simulink model "CCR_DIAM4100_model"  (R2023a)
settings: Solver=FixedStepAuto  StartTime=0.0  StopTime=1  RelTol=1e-3
values from neighbouring files (symbols this model uses):
  DIAM4100 = evalin('base', 'DIAM4100')    [DIAM4100_applyModelParameters.m]    (also in DIAM4100_simParams.m = cfg; DIAM4100_tuneKiSweep.m; DIAM4100_validateControl.m)
undefined symbols (not defined in the file or in its folder): D1, lagging, pulse
libraries: spsThyristorLib x2, spsACVoltageSourceLib x1, spsCurrentMeasurementLib x1, slpidlib x1, spsLinearTransformerLib x1, spsPLLLib x1, spsPulseGeneratorThyristor6PulseLib x1, spsRMSLib x1, spsSeriesRLCBranchLib x1, spsVoltageMeasurementLib x1, sps_lib x1
settings Model: Creator=KSSS  LastModifiedBy=KSSS

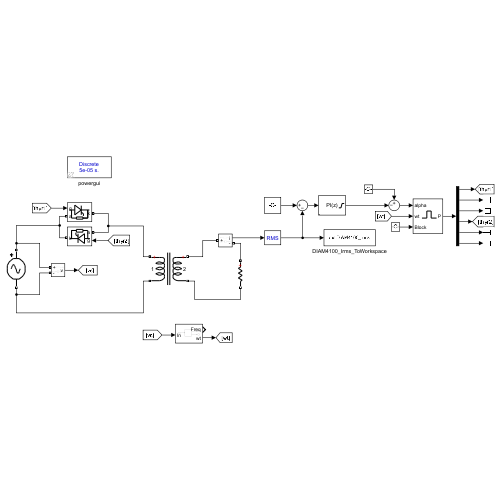
[thumbnail: Simulink's stored preview of the top-level diagram]
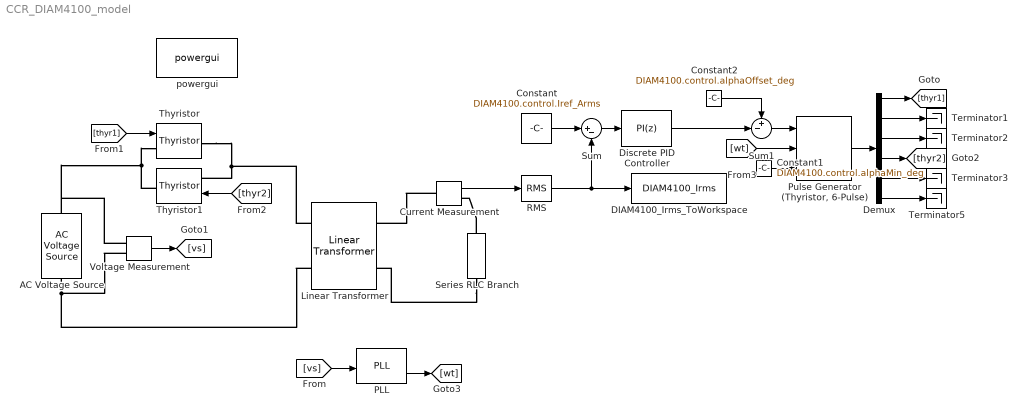
== system CCR_DIAM4100_model ==
  AC Voltage Source : spsACVoltageSourceLib/AC Voltage Source  Amplitude=DIAM4100.grid.Vpk  Phase=0  Frequency=DIAM4100.grid.f_Hz  SampleTime=0  Measurements=None  BusType=swing  Pref=10e3  Qref=0  Qmin=-inf  Qmax=+inf
  Constant : Constant  Value=DIAM4100.control.Iref_Arms
  Constant1 : Constant  Value=DIAM4100.control.alphaMin_deg
  Constant2 : Constant  Value=DIAM4100.control.alphaOffset_deg
  Current Measurement : spsCurrentMeasurementLib/Current Measurement  PhasorSimulation=off  OutputType=Complex  PSBequivalent=0
  DIAM4100_Irms_ToWorkspace : ToWorkspace  VariableName=DIAM4100_Irms  SaveFormat=Timeseries  SampleTime=-1
  Demux : Demux  Outputs=6
  Discrete PID Controller : slpidlib/PID Controller  Controller=PI  Form=Parallel  TimeDomain=Discrete-time  UseExternalTs=off  SampleTime=DIAM4100.control.Ts_s  IntegratorMethod=Forward Euler  FilterMethod=Forward Euler  ControllerParametersSource=internal  P=DIAM4100.control.Kp  I=DIAM4100.control.Ki  UseKiTs=off  D=0  N=100  UseFilter=on  TunerSelectOption=Transfer Function Based (PID Tuner App)  InitialConditionSource=internal  InitialConditionForIntegrator=DIAM4100.control.integratorIC_deg  InitialConditionForFilter=0  DifferentiatorICPrevScaledInput=0  ExternalReset=none  TrackingMode=off  Kt=1  LimitOutput=on  SatLimitsSource=internal  UpperSaturationLimit=DIAM4100.control.alphaMax_deg  LowerSaturationLimit=DIAM4100.control.alphaMin_deg  LinearizeAsGain=off  AntiWindupMode=clamping  Kb=1  LimitIntegrator=off  UpperIntegratorSaturationLimit=inf  LowerIntegratorSaturationLimit=-inf  RndMeth=Zero  POutMin=[]  POutMax=[]  IOutMin=[]  IOutMax=[]  DOutMin=[]  DOutMax=[]  NOutMin=[]  NOutMax=[]  SumOutMin=[]  SumOutMax=[]  SaturationOutMin=[]  SaturationOutMax=[]  PParamMin=[]  PParamMax=[]  IParamMin=[]  IParamMax=[]  DParamMin=[]  DParamMax=[]  NParamMin=[]  NParamMax=[]  KbParamMin=[]  KbParamMax=[]  KtParamMin=[]  KtParamMax=[]  KbOutMin=[]  KbOutMax=[]  KtOutMin=[]  KtOutMax=[]  IntegratorOutMin=[]  IntegratorOutMax=[]  FilterOutMin=[]  FilterOutMax=[]  SumI1OutMin=[]  SumI1OutMax=[]  SumI2OutMin=[]  SumI2OutMax=[]  SumI3OutMin=[]  SumI3OutMax=[]  SumI4OutMin=[]  SumI4OutMax=[]  SumDOutMin=[]  SumDOutMax=[]  DifferentiatorOutMin=[]  DifferentiatorOutMax=[]  FilterDiffOutCoefMin=[]  FilterDiffOutCoefMax=[]  ReciprocalOutMin=[]  ReciprocalOutMax=[]  SumDenOutMin=[]  SumDenOutMax=[]  SumNumOutMin=[]  SumNumOutMax=[]  DivideOutMin=[]  DivideOutMax=[]  UdiffTsProdOutMin=[]  UdiffTsProdOutMax=[]  NTsProdOutMin=[]  NTsProdOutMax=[]  UintegralTsProdOutMin=[]  UintegralTsProdOutMax=[]  UngainTsProdOutMin=[]  UngainTsProdOutMax=[]  ClampingZeroOutDataTypeStr=Inherit: Inherit via back propagation  ClampingZeroOutMin=[]  ClampingZeroOutMax=[]  FilterDenConstantOutDataTypeStr=Inherit: Inherit via back propagation  FilterDenConstantOutMin=[]  FilterDenConstantOutMax=[]  PCopyOutDataTypeStr=Inherit: Inherit via back propagation  PCopyOutMin=[]  PCopyOutMax=[]  NCopyOutDataTypeStr=Inherit: Inherit via back propagation  NCopyOutMin=[]  NCopyOutMax=[]  IntegratorContinuousStateAttributes=''  IntegratorStateMustResolveToSignalObject=off  IntegratorRTWStateStorageClass=Auto  FilterContinuousStateAttributes=''  FilterStateMustResolveToSignalObject=off  FilterRTWStateStorageClass=Auto  ParallelPVariant=InternalParameters  IdealPVariant=Disabled  IVariant=InternalParameters  DVariant=Disabled  IntegratorVariant=Discrete  SatVariant=Enabled  AWVariant=DiscClampingParallel  PCopyVariant=Disabled  TRVariant=Disabled  FdbkBlocksVariant=Forward  IdealPFdbkVariant=Disabled  SatFdbkVariant=Disabled  DerivativeFilterVariant=Disabled  NVariant=Disabled  NCopyVariant=Disabled_SignalSpec  FilterICVariant=Disabled  IntegratorICVariant=InternalICs  ExternalResetVariant=Disabled  TRSumVariant=Passthrough  SumFdbkVariant=Disabled  SumVariant=Sum_PI  TsampFilterVariant=InternalTs  TsampNgainVariant=Passthrough  TsampIntegralVariant=Disabled_SignalSpec  ExternalSaturationOutDataTypeStr=Inherit: Same as second input
      settings: LibrarySourceBlock=simulink/Discrete/Discrete PID Controller
  Linear Transformer : spsLinearTransformerLib/Linear Transformer  UNITS=pu  NominalPower=DIAM4100.transformer.NominalPower  winding1=DIAM4100.transformer.winding1  winding2=DIAM4100.transformer.winding2  ThreeWindings=off  winding3=[ 315e3 0.002 0.08 ]  RmLm=DIAM4100.transformer.RmLm  Measurements=None  DataType=off
  PLL : spsPLLLib/PLL  Fmin=45  Par_Init=[0 DIAM4100.grid.f_Hz]  ParK=[180, 3200, 1]  TcD=DIAM4100.control.Ts_s  MaxRateChangeFreq=12  FilterCutOffFreq=25  Ts=0  AGC=on
      settings: LibrarySourceBlock=sps_lib/Control/PLL
  "Pulse Generator (Thyristor, 6-Pulse)" : spsPulseGeneratorThyristor6PulseLib/Pulse Generator (Thyristor, 6-Pulse)  GenType=6-pulse  Delta=D1 (lagging)  pwidth=DIAM4100.pulse.pwidth_deg  Double_Pulse=off  Ts=DIAM4100.control.Ts_s
      settings: LibrarySourceBlock=|
      | sps_lib/Power Electronics/Power Electronics Control/Pulse Generator
      | (Thyristor, 6-Pulse)
  RMS : spsRMSLib/RMS  TrueRMS=on  Freq=DIAM4100.grid.f_Hz  RMSInit=0  Ts=0
  Series RLC Branch : spsSeriesRLCBranchLib/Series RLC Branch  LConnTagsString=__new0  RConnTagsString=__new0  BranchType=R  Resistance=DIAM4100.load.R_ohm  Inductance=DIAM4100.load.L_H  SetiL0=off  InitialCurrent=0  Capacitance=DIAM4100.load.C_F  Setx0=off  InitialVoltage=0  Measurements=None
  Sum : Sum  Inputs=|+-
  Sum1 : Sum  Inputs=+-|
  Terminator{1..3,5} (4 alike) : Terminator
  Thyristor : spsThyristorLib/Thyristor  Ron=DIAM4100.thyristor.Ron_ohm  Lon=DIAM4100.thyristor.Lon_H  Vf=DIAM4100.thyristor.Vf_V  IC=0  Rs=DIAM4100.thyristor.Rs_ohm  Cs=DIAM4100.thyristor.Cs_F  Measurements=off
  Thyristor1 : spsThyristorLib/Thyristor  Ron=DIAM4100.thyristor.Ron_ohm  Lon=DIAM4100.thyristor.Lon_H  Vf=DIAM4100.thyristor.Vf_V  IC=0  Rs=DIAM4100.thyristor.Rs_ohm  Cs=DIAM4100.thyristor.Cs_F  Measurements=off
  Voltage Measurement : spsVoltageMeasurementLib/Voltage Measurement  PhasorSimulation=off  OutputType=Complex  PSBequivalent=0
  powergui : sps_lib/powergui  Priority=1  SimulationMode=Discrete  SampleTime=DIAM4100.powergui.Ts_s  frequency=DIAM4100.grid.f_Hz  Iterations=50  frequencyindice=DIAM4100.grid.f_Hz  Pbase=100e6  ErrMax=1e-4  UnitsV=kV  UnitsW=MW  buscounter=0  FunctionMessages=off  echomessages=off  EnableUseOfTLC=off  CurrentSourceSwitches=off  DisableSnubberDevices=off  DisableRonSwitches=off  DisableVfSwitches=off  DisplayEquations=off  AutomaticDiscreteSolvers=off  SolverType=Tustin/Backward Euler (TBE)  Interpol=off  ExternalGateDelay=off  methode=off  Ts=100  x0status=blocks  SPID=on  SwTol=0  HookPort=off  NonlinearTolerance=1e-4  nMaxIteration=100  ContinueOnMaxIteration=off  RestoreLinks=warning  ResistiveCurrentMeasurement=off  Frange=[0:2:500]  Ylog=off  Xlog=on  ShowGrid=off  save=off  variable=ZData  structure=0  ZoomFFT=off  StartTime=0.0  cycles=1  DisplayStyle=1  fundamental=DIAM4100.grid.f_Hz  FreqAxis=off  MaxFrequency=1000  frequencyindicesteady=1  RmsSteady=1  display=off
  wires:
  Current Measurement/1 -> RMS/1
  Constant/1 -> Sum/1
  Sum/1 -> Discrete PID Controller/1
  [vs] -> PLL/1
  Voltage Measurement/1 -> [vs]
  Constant1/1 -> "Pulse Generator (Thyristor, 6-Pulse)"/3
  [thyr1] -> Thyristor/1
  [thyr2] -> Thyristor1/1
  Demux/1 -> [thyr1]
  [wt] -> "Pulse Generator (Thyristor, 6-Pulse)"/2
  PLL/2 -> [wt]
  "Pulse Generator (Thyristor, 6-Pulse)"/1 -> Demux/1
  Demux/4 -> [thyr2]
  Demux/2 -> Terminator1/1
  Demux/3 -> Terminator2/1
  Demux/5 -> Terminator3/1
  Demux/6 -> Terminator5/1
  Sum1/1 -> "Pulse Generator (Thyristor, 6-Pulse)"/1
  Discrete PID Controller/1 -> Sum1/2
  Constant2/1 -> Sum1/1
  RMS/1 -> Sum/2, DIAM4100_Irms_ToWorkspace/1
  connections:
  Thyristor/RConn1 -- Linear Transformer/LConn1 -- Thyristor1/LConn1
  Thyristor1/RConn1 -- Voltage Measurement/LConn1 -- AC Voltage Source/RConn1 -- Thyristor/LConn1
  Series RLC Branch/LConn1 -- Current Measurement/RConn1
  Voltage Measurement/LConn2 -- Linear Transformer/LConn2 -- AC Voltage Source/LConn1
  Series RLC Branch/RConn1 -- Linear Transformer/RConn2
  Current Measurement/LConn1 -- Linear Transformer/RConn1
